simulink model "average_linear_model_r2018b"  (R2018b)
settings: Solver=VariableStepAuto  StartTime=0.0  StopTime=10.0  RelTol=1e-3
undefined symbols (not defined in the file): D_COUNTER, D_ENABLED, D_LAST_INPUT, D_LAST_OUTPUT, D_LASTOUT_TIME, D_LASTTIME, D_NEXTTIME, D_SUM_TIME, DWORK_NUMBER
settings Model: Creator=jogo1652  LastModifiedBy=drhf
settings DataIOCC: ReturnWorkspaceOutputs=on

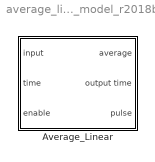
== system average_linear_model_r2018b ==
  Average_Linear : Subsystem  mask{time_intervall=3600, offset_flag=off, enable_flag=off}
      mask prompts: time_intervall "Delta_t"; offset_flag "start calculating every full hour"; enable_flag "only calculate when enabled"
      mask help:
      | This block calculates the average of each input vector during a specified time Delta_t. During this time interval the output is held.
      | The output time is the time of the last average calculation.
      | Every time the average is calculated again, a signal pulse of 1 is put out.
      |
      | When the full hour flag is set, the calculation of the average is started every full hour once again.
      |
      | When the enable flag is set, the functions calculates only while the enable signal is 1. When it is 0, the function repeats putting out the last output.
      mask init:
      | if time_intervall==0
      |     delta_t = 1;
      | else
      |     delta_t = time_intervall;
      | end
      mask Help: web(fullfile(path_carnot('help'),'Average.html'),'-helpbrowser')

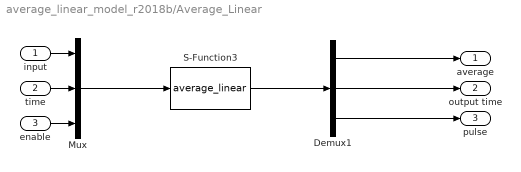
== system average_linear_model_r2018b/Average_Linear ==
  input : Inport
  time : Inport  Port=2
  enable : Inport  Port=3
  Demux1 : Demux  Outputs=[-1 1 1]
      settings: DisplayOption=none
  Mux : Mux  Inputs=3
  S-Function3 : S-Function  FunctionName=average_linear  Parameters=delta_t offset_flag enable_flag  SFunctionDeploymentMode=off  EnableBusSupport=off  SFcnStateName=D_LAST_OUTPUT,D_COUNTER,D_SUM_TIME,D_NEXTTIME,D_LASTTIME,D_LASTOUT_TIME,D_ENABLED,DWORK_NUMBER,D_LAST_INPUT
      settings: SFcnIsStateOwnerBlock=on
  average : Outport  VectorParamsAs1DForOutWhenUnconnected=off
  output time : Outport  Port=2  VectorParamsAs1DForOutWhenUnconnected=off
  pulse : Outport  Port=3  VectorParamsAs1DForOutWhenUnconnected=off
  wires:
  Mux/1 -> S-Function3/1
  enable/1 -> Mux/3
  input/1 -> Mux/1
  S-Function3/1 -> Demux1/1
  Demux1/2 -> output time/1
  time/1 -> Mux/2
  Demux1/3 -> pulse/1
  Demux1/1 -> average/1
